simulink model "ddc_bpm_476_066"  (Simulink 7.8)
settings: Solver=ode45  StartTime=0.0  StopTime=2e-3  RelTol=1e-3
undefined symbols (not defined in the file): decim_factor_poly_35, dt_sim, frev_476, Fs_adc, n_ch, n_ovs, R_fofb, R_sec, R_sec_cfir, R_sec_pfir, xlipgetpartsetting
libraries: xbsIndex_r4 x1491, simulink x7
(part 7 of 12)

== system ddc_bpm_476_066/delta-sigma_monit/downsample8 ==
  din : Inport
  Down Sample : xbsIndex_r4/Down Sample  sample_ratio=R_fofb*R_sec_cfir*R_sec_pfir  sample_phase="Last Value of Frame  (most efficient)"  en=off  latency=1  dbl_ovrd=off  block_type=dsamp
  Down Sample5 : xbsIndex_r4/Down Sample  sample_ratio=R_sec*n_ovs  sample_phase="Last Value of Frame  (most efficient)"  en=off  latency=1  dbl_ovrd=off  block_type=dsamp
  dout : Outport
  wires:
  Down Sample5/1 -> Down Sample/1
  Down Sample/1 -> dout/1
  din/1 -> Down Sample5/1

== system ddc_bpm_476_066/delta-sigma_monit/fifo_tbt_q ==
  din : Inport
  re : Inport  Port=2
  we : Inport  Port=3
  clr_vld : Inport  Port=4
  From FIFO : xbsIndex_r4/From FIFO  shared_memory_name='fifo_monit_ds_q'  ownership=Owned elsewhere  performance_options=Standard_FIFO  depth=16  percent_nbits=1  has_arst=off  use_percent_full_port=off  gui_display_data_type=Fixed-point  arith_type="Signed  (2's comp)"  n_bits=26  bin_pt=22  preci_type=Single  dbl_ovrd=off  mem_type=Distributed RAM  block_type=fromfifo
      settings: AttributesFormatString=<< %<shared_memory_name> >>  infoedit=First-in-first-out (FIFO) block that reads FIFO data from shared memory storage.
  Inverter2 : xbsIndex_r4/Inverter  en=off  latency=0  dbl_ovrd=off  block_type=inv
  Inverter4 : xbsIndex_r4/Inverter  en=off  latency=0  dbl_ovrd=off  block_type=inv
  Logical : xbsIndex_r4/Logical  logical_function=AND  inputs=2  en=off  latency=0  precision=Full  arith_type=Unsigned  n_bits=16  bin_pt=0  align_bp=on  dbl_ovrd=off  block_type=logical
  Logical2 : xbsIndex_r4/Logical  logical_function=AND  inputs=2  en=off  latency=0  precision=Full  arith_type=Unsigned  n_bits=16  bin_pt=0  align_bp=on  dbl_ovrd=off  block_type=logical
  Register : xbsIndex_r4/Register  init=0  rst=off  en=off  dbl_ovrd=off  block_type=register
  ST11 : Subsystem
  ST2 : Subsystem
  ST7 : Subsystem
  To FIFO : xbsIndex_r4/To FIFO  shared_memory_name='fifo_monit_ds_q'  ownership=Locally owned  performance_options=Standard_FIFO  depth=16  percent_nbits=1  has_arst=off  use_percent_full_port=off  explicit_data_type=off  gui_display_data_type=Fixed-point  arith_type="Signed  (2's comp)"  n_bits=16  bin_pt=14  preci_type=Single  dbl_ovrd=off  mem_type=Distributed RAM  block_type=tofifo
      settings: AttributesFormatString=<< %<shared_memory_name> >>  infoedit=First-in-first-out (FIFO) block that writes FIFO data to shared memory storage.
  pulse_stretcher : Subsystem
  dout : Outport
  wr_full : Outport  Port=2
  rd_empty : Outport  Port=3
  valid_out : Outport  Port=4
  wires:
  Inverter2/1 -> Logical/2
  Logical/1 -> To FIFO/2, ST11/1(In)  "we"
  To FIFO/1 -> Inverter2/1, wr_full/1  "full"
  From FIFO/1 -> dout/1, ST2/1(In)  "dividend_data"
  we/1 -> Logical/1
  din/1 -> To FIFO/1
  From FIFO/2 -> rd_empty/1, Inverter4/1  "empty"
  clr_vld/1 -> pulse_stretcher/2(clr)  "clr"
  Register/1 -> pulse_stretcher/1(pulse_in)
  pulse_stretcher/1(extd_out) -> valid_out/1
  re/1 -> Logical2/1, ST7/1(In)
  Logical2/1 -> From FIFO/1, Register/1
  Inverter4/1 -> Logical2/2  "dividend_valid"

== system ddc_bpm_476_066/delta-sigma_monit/fifo_tbt_sum ==
  din : Inport
  re : Inport  Port=2
  we : Inport  Port=3
  clr_vld : Inport  Port=4
  From FIFO : xbsIndex_r4/From FIFO  shared_memory_name='fifo_monit_ds_sum'  ownership=Owned elsewhere  performance_options=Standard_FIFO  depth=16  percent_nbits=1  has_arst=off  use_percent_full_port=off  gui_display_data_type=Fixed-point  arith_type="Signed  (2's comp)"  n_bits=26  bin_pt=22  preci_type=Single  dbl_ovrd=off  mem_type=Distributed RAM  block_type=fromfifo
      settings: AttributesFormatString=<< %<shared_memory_name> >>  infoedit=First-in-first-out (FIFO) block that reads FIFO data from shared memory storage.
  Inverter2 : xbsIndex_r4/Inverter  en=off  latency=0  dbl_ovrd=off  block_type=inv
  Inverter4 : xbsIndex_r4/Inverter  en=off  latency=0  dbl_ovrd=off  block_type=inv
  Logical : xbsIndex_r4/Logical  logical_function=AND  inputs=2  en=off  latency=0  precision=Full  arith_type=Unsigned  n_bits=16  bin_pt=0  align_bp=on  dbl_ovrd=off  block_type=logical
  Logical2 : xbsIndex_r4/Logical  logical_function=AND  inputs=2  en=off  latency=0  precision=Full  arith_type=Unsigned  n_bits=16  bin_pt=0  align_bp=on  dbl_ovrd=off  block_type=logical
  Register : xbsIndex_r4/Register  init=0  rst=off  en=off  dbl_ovrd=off  block_type=register
  ST11 : Subsystem
  ST2 : Subsystem
  ST7 : Subsystem
  To FIFO : xbsIndex_r4/To FIFO  shared_memory_name='fifo_monit_ds_sum'  ownership=Locally owned  performance_options=Standard_FIFO  depth=16  percent_nbits=1  has_arst=off  use_percent_full_port=off  explicit_data_type=off  gui_display_data_type=Fixed-point  arith_type="Signed  (2's comp)"  n_bits=16  bin_pt=14  preci_type=Single  dbl_ovrd=off  mem_type=Distributed RAM  block_type=tofifo
      settings: AttributesFormatString=<< %<shared_memory_name> >>  infoedit=First-in-first-out (FIFO) block that writes FIFO data to shared memory storage.
  pulse_stretcher : Subsystem
  dout : Outport
  wr_full : Outport  Port=2
  rd_empty : Outport  Port=3
  valid_out : Outport  Port=4
  wires:
  Inverter2/1 -> Logical/2
  Logical/1 -> To FIFO/2, ST11/1(In)  "we"
  To FIFO/1 -> Inverter2/1, wr_full/1  "full"
  From FIFO/1 -> dout/1, ST2/1(In)  "dividend_data"
  we/1 -> Logical/1
  din/1 -> To FIFO/1
  From FIFO/2 -> rd_empty/1, Inverter4/1  "empty"
  clr_vld/1 -> pulse_stretcher/2(clr)  "clr"
  Register/1 -> pulse_stretcher/1(pulse_in)
  pulse_stretcher/1(extd_out) -> valid_out/1
  re/1 -> Logical2/1, ST7/1(In)
  Logical2/1 -> From FIFO/1, Register/1
  Inverter4/1 -> Logical2/2  "dividend_valid"

== system ddc_bpm_476_066/delta-sigma_monit/fifo_tbt_x ==
  din : Inport
  re : Inport  Port=2
  we : Inport  Port=3
  clr_vld : Inport  Port=4
  From FIFO : xbsIndex_r4/From FIFO  shared_memory_name='fifo_monit_ds_x'  ownership=Owned elsewhere  performance_options=Standard_FIFO  depth=16  percent_nbits=1  has_arst=off  use_percent_full_port=off  gui_display_data_type=Fixed-point  arith_type="Signed  (2's comp)"  n_bits=26  bin_pt=22  preci_type=Single  dbl_ovrd=off  mem_type=Distributed RAM  block_type=fromfifo
      settings: AttributesFormatString=<< %<shared_memory_name> >>  infoedit=First-in-first-out (FIFO) block that reads FIFO data from shared memory storage.
  Inverter2 : xbsIndex_r4/Inverter  en=off  latency=0  dbl_ovrd=off  block_type=inv
  Inverter4 : xbsIndex_r4/Inverter  en=off  latency=0  dbl_ovrd=off  block_type=inv
  Logical : xbsIndex_r4/Logical  logical_function=AND  inputs=2  en=off  latency=0  precision=Full  arith_type=Unsigned  n_bits=16  bin_pt=0  align_bp=on  dbl_ovrd=off  block_type=logical
  Logical2 : xbsIndex_r4/Logical  logical_function=AND  inputs=2  en=off  latency=0  precision=Full  arith_type=Unsigned  n_bits=16  bin_pt=0  align_bp=on  dbl_ovrd=off  block_type=logical
  Register : xbsIndex_r4/Register  init=0  rst=off  en=off  dbl_ovrd=off  block_type=register
  ST11 : Subsystem
  ST2 : Subsystem
  ST7 : Subsystem
  To FIFO : xbsIndex_r4/To FIFO  shared_memory_name='fifo_monit_ds_x'  ownership=Locally owned  performance_options=Standard_FIFO  depth=16  percent_nbits=1  has_arst=off  use_percent_full_port=off  explicit_data_type=off  gui_display_data_type=Fixed-point  arith_type="Signed  (2's comp)"  n_bits=16  bin_pt=14  preci_type=Single  dbl_ovrd=off  mem_type=Distributed RAM  block_type=tofifo
      settings: AttributesFormatString=<< %<shared_memory_name> >>  infoedit=First-in-first-out (FIFO) block that writes FIFO data to shared memory storage.
  pulse_stretcher : Subsystem
  dout : Outport
  wr_full : Outport  Port=2
  rd_empty : Outport  Port=3
  valid_out : Outport  Port=4
  wires:
  Inverter2/1 -> Logical/2
  Logical/1 -> To FIFO/2, ST11/1(In)  "we"
  To FIFO/1 -> Inverter2/1, wr_full/1  "full"
  From FIFO/1 -> dout/1, ST2/1(In)  "dividend_data"
  we/1 -> Logical/1
  din/1 -> To FIFO/1
  From FIFO/2 -> rd_empty/1, Inverter4/1  "empty"
  clr_vld/1 -> pulse_stretcher/2(clr)  "clr"
  Register/1 -> pulse_stretcher/1(pulse_in)
  pulse_stretcher/1(extd_out) -> valid_out/1
  re/1 -> Logical2/1, ST7/1(In)
  Logical2/1 -> From FIFO/1, Register/1
  Inverter4/1 -> Logical2/2  "dividend_valid"

== system ddc_bpm_476_066/delta-sigma_monit/fifo_tbt_y ==
  din : Inport
  re : Inport  Port=2
  we : Inport  Port=3
  clr_vld : Inport  Port=4
  From FIFO : xbsIndex_r4/From FIFO  shared_memory_name='fifo_monit_ds_y'  ownership=Owned elsewhere  performance_options=Standard_FIFO  depth=16  percent_nbits=1  has_arst=off  use_percent_full_port=off  gui_display_data_type=Fixed-point  arith_type="Signed  (2's comp)"  n_bits=26  bin_pt=22  preci_type=Single  dbl_ovrd=off  mem_type=Distributed RAM  block_type=fromfifo
      settings: AttributesFormatString=<< %<shared_memory_name> >>  infoedit=First-in-first-out (FIFO) block that reads FIFO data from shared memory storage.
  Inverter2 : xbsIndex_r4/Inverter  en=off  latency=0  dbl_ovrd=off  block_type=inv
  Inverter4 : xbsIndex_r4/Inverter  en=off  latency=0  dbl_ovrd=off  block_type=inv
  Logical : xbsIndex_r4/Logical  logical_function=AND  inputs=2  en=off  latency=0  precision=Full  arith_type=Unsigned  n_bits=16  bin_pt=0  align_bp=on  dbl_ovrd=off  block_type=logical
  Logical2 : xbsIndex_r4/Logical  logical_function=AND  inputs=2  en=off  latency=0  precision=Full  arith_type=Unsigned  n_bits=16  bin_pt=0  align_bp=on  dbl_ovrd=off  block_type=logical
  Register : xbsIndex_r4/Register  init=0  rst=off  en=off  dbl_ovrd=off  block_type=register
  ST11 : Subsystem
  ST2 : Subsystem
  ST7 : Subsystem
  To FIFO : xbsIndex_r4/To FIFO  shared_memory_name='fifo_monit_ds_y'  ownership=Locally owned  performance_options=Standard_FIFO  depth=16  percent_nbits=1  has_arst=off  use_percent_full_port=off  explicit_data_type=off  gui_display_data_type=Fixed-point  arith_type="Signed  (2's comp)"  n_bits=16  bin_pt=14  preci_type=Single  dbl_ovrd=off  mem_type=Distributed RAM  block_type=tofifo
      settings: AttributesFormatString=<< %<shared_memory_name> >>  infoedit=First-in-first-out (FIFO) block that writes FIFO data to shared memory storage.
  WaveScope : xbsIndex_r4/WaveScope  block_type=wavescope
  pulse_stretcher : Subsystem
  dout : Outport
  wr_full : Outport  Port=2
  rd_empty : Outport  Port=3
  valid_out : Outport  Port=4
  wires:
  Inverter2/1 -> Logical/2
  Logical/1 -> To FIFO/2, ST11/1(In)  "we"
  To FIFO/1 -> Inverter2/1, wr_full/1  "full"
  From FIFO/1 -> dout/1, ST2/1(In)  "dividend_data"
  we/1 -> Logical/1
  din/1 -> To FIFO/1
  From FIFO/2 -> rd_empty/1, Inverter4/1  "empty"
  clr_vld/1 -> pulse_stretcher/2(clr)  "clr"
  Register/1 -> pulse_stretcher/1(pulse_in)  "re_and_dly"
  pulse_stretcher/1(extd_out) -> valid_out/1  "vld_out"
  re/1 -> Logical2/1, ST7/1(In)  "re"
  Logical2/1 -> Register/1, From FIFO/1  "re_and"
  Inverter4/1 -> Logical2/2  "no_empty"

== system ddc_bpm_476_066/delta-sigma_monit/pulse_stretcher ==
  pulse_in : Inport
  clr : Inport  Port=2
  Inverter : xbsIndex_r4/Inverter  en=off  latency=0  dbl_ovrd=off  block_type=inv
  Logical1 : xbsIndex_r4/Logical  logical_function=AND  inputs=2  en=off  latency=0  precision=Full  arith_type=Unsigned  n_bits=16  bin_pt=0  align_bp=on  dbl_ovrd=off  block_type=logical
  Logical2 : xbsIndex_r4/Logical  logical_function=OR  inputs=2  en=off  latency=0  precision=Full  arith_type=Unsigned  n_bits=16  bin_pt=0  align_bp=on  dbl_ovrd=off  block_type=logical
  Logical3 : xbsIndex_r4/Logical  logical_function=OR  inputs=2  en=off  latency=0  precision=Full  arith_type=Unsigned  n_bits=16  bin_pt=0  align_bp=on  dbl_ovrd=off  block_type=logical
  Register : xbsIndex_r4/Register  init=0  rst=off  en=off  dbl_ovrd=off  block_type=register
  extd_out : Outport
  wires:
  Register/1 -> Logical1/1, Logical3/2
  clr/1 -> Inverter/1
  Logical1/1 -> Logical2/2
  Logical2/1 -> Register/1
  Inverter/1 -> Logical1/2
  Logical3/1 -> extd_out/1
  pulse_in/1 -> Logical3/1, Logical2/1

== system ddc_bpm_476_066/delta-sigma_monit/pulse_stretcher1 ==
  pulse_in : Inport
  clr : Inport  Port=2
  Inverter : xbsIndex_r4/Inverter  en=off  latency=0  dbl_ovrd=off  block_type=inv
  Logical1 : xbsIndex_r4/Logical  logical_function=AND  inputs=2  en=off  latency=0  precision=Full  arith_type=Unsigned  n_bits=16  bin_pt=0  align_bp=on  dbl_ovrd=off  block_type=logical
  Logical2 : xbsIndex_r4/Logical  logical_function=OR  inputs=2  en=off  latency=0  precision=Full  arith_type=Unsigned  n_bits=16  bin_pt=0  align_bp=on  dbl_ovrd=off  block_type=logical
  Logical3 : xbsIndex_r4/Logical  logical_function=OR  inputs=2  en=off  latency=0  precision=Full  arith_type=Unsigned  n_bits=16  bin_pt=0  align_bp=on  dbl_ovrd=off  block_type=logical
  Register : xbsIndex_r4/Register  init=0  rst=off  en=off  dbl_ovrd=off  block_type=register
  extd_out : Outport
  wires:
  Register/1 -> Logical1/1, Logical3/2
  clr/1 -> Inverter/1
  Logical1/1 -> Logical2/2
  Logical2/1 -> Register/1
  Inverter/1 -> Logical1/2
  Logical3/1 -> extd_out/1
  pulse_in/1 -> Logical3/1, Logical2/1

== system ddc_bpm_476_066/delta-sigma_monit/pulse_stretcher2 ==
  pulse_in : Inport
  clr : Inport  Port=2
  Inverter : xbsIndex_r4/Inverter  en=off  latency=0  dbl_ovrd=off  block_type=inv
  Logical1 : xbsIndex_r4/Logical  logical_function=AND  inputs=2  en=off  latency=0  precision=Full  arith_type=Unsigned  n_bits=16  bin_pt=0  align_bp=on  dbl_ovrd=off  block_type=logical
  Logical2 : xbsIndex_r4/Logical  logical_function=OR  inputs=2  en=off  latency=0  precision=Full  arith_type=Unsigned  n_bits=16  bin_pt=0  align_bp=on  dbl_ovrd=off  block_type=logical
  Logical3 : xbsIndex_r4/Logical  logical_function=OR  inputs=2  en=off  latency=0  precision=Full  arith_type=Unsigned  n_bits=16  bin_pt=0  align_bp=on  dbl_ovrd=off  block_type=logical
  Register : xbsIndex_r4/Register  init=0  rst=off  en=off  dbl_ovrd=off  block_type=register
  extd_out : Outport
  wires:
  Register/1 -> Logical1/1, Logical3/2
  clr/1 -> Inverter/1
  Logical1/1 -> Logical2/2
  Logical2/1 -> Register/1
  Inverter/1 -> Logical1/2
  Logical3/1 -> extd_out/1
  pulse_in/1 -> Logical3/1, Logical2/1

== system ddc_bpm_476_066/delta-sigma_monit/pulse_stretcher3 ==
  pulse_in : Inport
  clr : Inport  Port=2
  Inverter : xbsIndex_r4/Inverter  en=off  latency=0  dbl_ovrd=off  block_type=inv
  Logical1 : xbsIndex_r4/Logical  logical_function=AND  inputs=2  en=off  latency=0  precision=Full  arith_type=Unsigned  n_bits=16  bin_pt=0  align_bp=on  dbl_ovrd=off  block_type=logical
  Logical2 : xbsIndex_r4/Logical  logical_function=OR  inputs=2  en=off  latency=0  precision=Full  arith_type=Unsigned  n_bits=16  bin_pt=0  align_bp=on  dbl_ovrd=off  block_type=logical
  Logical3 : xbsIndex_r4/Logical  logical_function=OR  inputs=2  en=off  latency=0  precision=Full  arith_type=Unsigned  n_bits=16  bin_pt=0  align_bp=on  dbl_ovrd=off  block_type=logical
  Register : xbsIndex_r4/Register  init=0  rst=off  en=off  dbl_ovrd=off  block_type=register
  extd_out : Outport
  wires:
  Register/1 -> Logical1/1, Logical3/2
  clr/1 -> Inverter/1
  Logical1/1 -> Logical2/2
  Logical2/1 -> Register/1
  Inverter/1 -> Logical1/2
  Logical3/1 -> extd_out/1
  pulse_in/1 -> Logical3/1, Logical2/1

== system ddc_bpm_476_066/delta-sigma_tbt/DataReg_En ==
  Din : Inport
  en : Inport  Port=2
  Register : xbsIndex_r4/Register  init=0  rst=off  en=on  dbl_ovrd=off  block_type=register
      settings: block_version=VER_STRING_GOES_HERE
  Register1 : xbsIndex_r4/Register  init=0  rst=off  en=off  dbl_ovrd=off  block_type=register
      settings: block_version=VER_STRING_GOES_HERE
  Dout : Outport
  Valid : Outport  Port=2
  wires:
  Din/1 -> Register/1
  Register/1 -> Dout/1
  Register1/1 -> Valid/1
  en/1 -> Register1/1, Register/2

== system ddc_bpm_476_066/delta-sigma_tbt/DataReg_En1 ==
  Din : Inport
  en : Inport  Port=2
  Register : xbsIndex_r4/Register  init=0  rst=off  en=on  dbl_ovrd=off  block_type=register
      settings: block_version=VER_STRING_GOES_HERE
  Register1 : xbsIndex_r4/Register  init=0  rst=off  en=off  dbl_ovrd=off  block_type=register
      settings: block_version=VER_STRING_GOES_HERE
  Dout : Outport
  Valid : Outport  Port=2
  wires:
  Din/1 -> Register/1
  Register/1 -> Dout/1
  Register1/1 -> Valid/1
  en/1 -> Register1/1, Register/2

== system ddc_bpm_476_066/delta-sigma_tbt/DataReg_En2 ==
  Din : Inport
  en : Inport  Port=2
  Register : xbsIndex_r4/Register  init=0  rst=off  en=on  dbl_ovrd=off  block_type=register
      settings: block_version=VER_STRING_GOES_HERE
  Register1 : xbsIndex_r4/Register  init=0  rst=off  en=off  dbl_ovrd=off  block_type=register
      settings: block_version=VER_STRING_GOES_HERE
  Dout : Outport
  Valid : Outport  Port=2
  wires:
  Din/1 -> Register/1
  Register/1 -> Dout/1
  Register1/1 -> Valid/1
  en/1 -> Register1/1, Register/2

== system ddc_bpm_476_066/delta-sigma_tbt/DataReg_En3 ==
  Din : Inport
  en : Inport  Port=2
  Register : xbsIndex_r4/Register  init=0  rst=off  en=on  dbl_ovrd=off  block_type=register
      settings: block_version=VER_STRING_GOES_HERE
  Register1 : xbsIndex_r4/Register  init=0  rst=off  en=off  dbl_ovrd=off  block_type=register
      settings: block_version=VER_STRING_GOES_HERE
  Dout : Outport
  Valid : Outport  Port=2
  wires:
  Din/1 -> Register/1
  Register/1 -> Dout/1
  Register1/1 -> Valid/1
  en/1 -> Register1/1, Register/2

== system ddc_bpm_476_066/delta-sigma_tbt/ST1 ==
  In : Inport
  Display : Display
  Sample Time : xbsIndex_r4/Sample Time  block_type=sampletime
      settings: infoedit="The Sample Time block reports the normalized sample period of its input.  A signal's normalized sample period is not equivalent to its Simulink absolute sample period.<br><br>Hardware notes: This block is implemented as a constant in hardware."
  X_monit1 : xbsIndex_r4/Gateway Out  inherit_from_input=on  hdl_port=off  timing_constraint=Data Rate  locs_specified=off  LOCs={}  UseAsDAC=off  DACChannel='1'  block_type=gatewayout
      settings: infoedit="Gateway out block.  Converts Xilinx fixed-point or floating-point type inputs into ouputs of type Simulink integer, single, double, or fixed point.<br><br>Hardware notes:  In hardware these blocks become top level output ports or are discarded, depending on how they are configured."
  wires:
  X_monit1/1 -> Display/1
  Sample Time/1 -> X_monit1/1
  In/1 -> Sample Time/1

== system ddc_bpm_476_066/delta-sigma_tbt/ST2 ==
  In : Inport
  Display : Display
  Sample Time : xbsIndex_r4/Sample Time  block_type=sampletime
      settings: infoedit="The Sample Time block reports the normalized sample period of its input.  A signal's normalized sample period is not equivalent to its Simulink absolute sample period.<br><br>Hardware notes: This block is implemented as a constant in hardware."
  X_monit1 : xbsIndex_r4/Gateway Out  inherit_from_input=on  hdl_port=off  timing_constraint=Data Rate  locs_specified=off  LOCs={}  UseAsDAC=off  DACChannel='1'  block_type=gatewayout
      settings: infoedit="Gateway out block.  Converts Xilinx fixed-point or floating-point type inputs into ouputs of type Simulink integer, single, double, or fixed point.<br><br>Hardware notes:  In hardware these blocks become top level output ports or are discarded, depending on how they are configured."
  wires:
  X_monit1/1 -> Display/1
  Sample Time/1 -> X_monit1/1
  In/1 -> Sample Time/1

== system ddc_bpm_476_066/delta-sigma_tbt/ST3 ==
  In : Inport
  Display : Display
  Sample Time : xbsIndex_r4/Sample Time  block_type=sampletime
      settings: infoedit="The Sample Time block reports the normalized sample period of its input.  A signal's normalized sample period is not equivalent to its Simulink absolute sample period.<br><br>Hardware notes: This block is implemented as a constant in hardware."
  X_monit1 : xbsIndex_r4/Gateway Out  inherit_from_input=on  hdl_port=off  timing_constraint=Data Rate  locs_specified=off  LOCs={}  UseAsDAC=off  DACChannel='1'  block_type=gatewayout
      settings: infoedit="Gateway out block.  Converts Xilinx fixed-point or floating-point type inputs into ouputs of type Simulink integer, single, double, or fixed point.<br><br>Hardware notes:  In hardware these blocks become top level output ports or are discarded, depending on how they are configured."
  wires:
  X_monit1/1 -> Display/1
  Sample Time/1 -> X_monit1/1
  In/1 -> Sample Time/1

== system ddc_bpm_476_066/delta-sigma_tbt/ST4 ==
  In : Inport
  Display : Display
  Sample Time : xbsIndex_r4/Sample Time  block_type=sampletime
      settings: infoedit="The Sample Time block reports the normalized sample period of its input.  A signal's normalized sample period is not equivalent to its Simulink absolute sample period.<br><br>Hardware notes: This block is implemented as a constant in hardware."
  X_monit1 : xbsIndex_r4/Gateway Out  inherit_from_input=on  hdl_port=off  timing_constraint=Data Rate  locs_specified=off  LOCs={}  UseAsDAC=off  DACChannel='1'  block_type=gatewayout
      settings: infoedit="Gateway out block.  Converts Xilinx fixed-point or floating-point type inputs into ouputs of type Simulink integer, single, double, or fixed point.<br><br>Hardware notes:  In hardware these blocks become top level output ports or are discarded, depending on how they are configured."
  wires:
  X_monit1/1 -> Display/1
  Sample Time/1 -> X_monit1/1
  In/1 -> Sample Time/1

== system ddc_bpm_476_066/delta-sigma_tbt/ST5 ==
  In : Inport
  Display : Display
  Sample Time : xbsIndex_r4/Sample Time  block_type=sampletime
      settings: infoedit="The Sample Time block reports the normalized sample period of its input.  A signal's normalized sample period is not equivalent to its Simulink absolute sample period.<br><br>Hardware notes: This block is implemented as a constant in hardware."
  X_monit1 : xbsIndex_r4/Gateway Out  inherit_from_input=on  hdl_port=off  timing_constraint=Data Rate  locs_specified=off  LOCs={}  UseAsDAC=off  DACChannel='1'  block_type=gatewayout
      settings: infoedit="Gateway out block.  Converts Xilinx fixed-point or floating-point type inputs into ouputs of type Simulink integer, single, double, or fixed point.<br><br>Hardware notes:  In hardware these blocks become top level output ports or are discarded, depending on how they are configured."
  wires:
  X_monit1/1 -> Display/1
  Sample Time/1 -> X_monit1/1
  In/1 -> Sample Time/1

== system ddc_bpm_476_066/delta-sigma_tbt/ST6 ==
  In : Inport
  Display : Display
  Sample Time : xbsIndex_r4/Sample Time  block_type=sampletime
      settings: infoedit="The Sample Time block reports the normalized sample period of its input.  A signal's normalized sample period is not equivalent to its Simulink absolute sample period.<br><br>Hardware notes: This block is implemented as a constant in hardware."
  X_monit1 : xbsIndex_r4/Gateway Out  inherit_from_input=on  hdl_port=off  timing_constraint=Data Rate  locs_specified=off  LOCs={}  UseAsDAC=off  DACChannel='1'  block_type=gatewayout
      settings: infoedit="Gateway out block.  Converts Xilinx fixed-point or floating-point type inputs into ouputs of type Simulink integer, single, double, or fixed point.<br><br>Hardware notes:  In hardware these blocks become top level output ports or are discarded, depending on how they are configured."
  wires:
  X_monit1/1 -> Display/1
  Sample Time/1 -> X_monit1/1
  In/1 -> Sample Time/1

== system ddc_bpm_476_066/delta-sigma_tbt/ST7 ==
  In : Inport
  Display : Display
  Sample Time : xbsIndex_r4/Sample Time  block_type=sampletime
      settings: infoedit="The Sample Time block reports the normalized sample period of its input.  A signal's normalized sample period is not equivalent to its Simulink absolute sample period.<br><br>Hardware notes: This block is implemented as a constant in hardware."
  X_monit1 : xbsIndex_r4/Gateway Out  inherit_from_input=on  hdl_port=off  timing_constraint=Data Rate  locs_specified=off  LOCs={}  UseAsDAC=off  DACChannel='1'  block_type=gatewayout
      settings: infoedit="Gateway out block.  Converts Xilinx fixed-point or floating-point type inputs into ouputs of type Simulink integer, single, double, or fixed point.<br><br>Hardware notes:  In hardware these blocks become top level output ports or are discarded, depending on how they are configured."
  wires:
  X_monit1/1 -> Display/1
  Sample Time/1 -> X_monit1/1
  In/1 -> Sample Time/1

== system ddc_bpm_476_066/delta-sigma_tbt/ST8 ==
  In : Inport
  Display : Display
  Sample Time : xbsIndex_r4/Sample Time  block_type=sampletime
      settings: infoedit="The Sample Time block reports the normalized sample period of its input.  A signal's normalized sample period is not equivalent to its Simulink absolute sample period.<br><br>Hardware notes: This block is implemented as a constant in hardware."
  X_monit1 : xbsIndex_r4/Gateway Out  inherit_from_input=on  hdl_port=off  timing_constraint=Data Rate  locs_specified=off  LOCs={}  UseAsDAC=off  DACChannel='1'  block_type=gatewayout
      settings: infoedit="Gateway out block.  Converts Xilinx fixed-point or floating-point type inputs into ouputs of type Simulink integer, single, double, or fixed point.<br><br>Hardware notes:  In hardware these blocks become top level output ports or are discarded, depending on how they are configured."
  wires:
  X_monit1/1 -> Display/1
  Sample Time/1 -> X_monit1/1
  In/1 -> Sample Time/1

== system ddc_bpm_476_066/delta-sigma_tbt/ST9 ==
  In : Inport
  Display : Display
  Sample Time : xbsIndex_r4/Sample Time  block_type=sampletime
      settings: infoedit="The Sample Time block reports the normalized sample period of its input.  A signal's normalized sample period is not equivalent to its Simulink absolute sample period.<br><br>Hardware notes: This block is implemented as a constant in hardware."
  X_monit1 : xbsIndex_r4/Gateway Out  inherit_from_input=on  hdl_port=off  timing_constraint=Data Rate  locs_specified=off  LOCs={}  UseAsDAC=off  DACChannel='1'  block_type=gatewayout
      settings: infoedit="Gateway out block.  Converts Xilinx fixed-point or floating-point type inputs into ouputs of type Simulink integer, single, double, or fixed point.<br><br>Hardware notes:  In hardware these blocks become top level output ports or are discarded, depending on how they are configured."
  wires:
  X_monit1/1 -> Display/1
  Sample Time/1 -> X_monit1/1
  In/1 -> Sample Time/1

== system ddc_bpm_476_066/delta-sigma_tbt/fifo_tbt_q ==
  din : Inport
  re : Inport  Port=2
  we : Inport  Port=3
  clr_vld : Inport  Port=4
  From FIFO : xbsIndex_r4/From FIFO  shared_memory_name='fifo_tbt_ds_q'  ownership=Owned elsewhere  performance_options=Standard_FIFO  depth=16  percent_nbits=1  has_arst=off  use_percent_full_port=off  gui_display_data_type=Fixed-point  arith_type="Signed  (2's comp)"  n_bits=26  bin_pt=22  preci_type=Single  dbl_ovrd=off  mem_type=Distributed RAM  block_type=fromfifo
      settings: AttributesFormatString=<< %<shared_memory_name> >>  infoedit=First-in-first-out (FIFO) block that reads FIFO data from shared memory storage.
  Inverter2 : xbsIndex_r4/Inverter  en=off  latency=0  dbl_ovrd=off  block_type=inv
  Inverter4 : xbsIndex_r4/Inverter  en=off  latency=0  dbl_ovrd=off  block_type=inv
  Logical : xbsIndex_r4/Logical  logical_function=AND  inputs=2  en=off  latency=0  precision=Full  arith_type=Unsigned  n_bits=16  bin_pt=0  align_bp=on  dbl_ovrd=off  block_type=logical
  Logical2 : xbsIndex_r4/Logical  logical_function=AND  inputs=2  en=off  latency=0  precision=Full  arith_type=Unsigned  n_bits=16  bin_pt=0  align_bp=on  dbl_ovrd=off  block_type=logical
  Register : xbsIndex_r4/Register  init=0  rst=off  en=off  dbl_ovrd=off  block_type=register
  ST11 : Subsystem
  ST2 : Subsystem
  ST7 : Subsystem
  To FIFO : xbsIndex_r4/To FIFO  shared_memory_name='fifo_tbt_ds_q'  ownership=Locally owned  performance_options=Standard_FIFO  depth=16  percent_nbits=1  has_arst=off  use_percent_full_port=off  explicit_data_type=off  gui_display_data_type=Fixed-point  arith_type="Signed  (2's comp)"  n_bits=16  bin_pt=14  preci_type=Single  dbl_ovrd=off  mem_type=Distributed RAM  block_type=tofifo
      settings: AttributesFormatString=<< %<shared_memory_name> >>  infoedit=First-in-first-out (FIFO) block that writes FIFO data to shared memory storage.
  pulse_stretcher : Subsystem
  dout : Outport
  wr_full : Outport  Port=2
  rd_empty : Outport  Port=3
  valid_out : Outport  Port=4
  wires:
  Inverter2/1 -> Logical/2
  Logical/1 -> To FIFO/2, ST11/1(In)  "we"
  To FIFO/1 -> Inverter2/1, wr_full/1  "full"
  From FIFO/1 -> dout/1, ST2/1(In)  "dividend_data"
  we/1 -> Logical/1
  din/1 -> To FIFO/1
  From FIFO/2 -> rd_empty/1, Inverter4/1  "empty"
  clr_vld/1 -> pulse_stretcher/2(clr)  "clr"
  Register/1 -> pulse_stretcher/1(pulse_in)
  pulse_stretcher/1(extd_out) -> valid_out/1
  re/1 -> Logical2/1, ST7/1(In)
  Logical2/1 -> From FIFO/1, Register/1
  Inverter4/1 -> Logical2/2  "dividend_valid"

== system ddc_bpm_476_066/delta-sigma_tbt/fifo_tbt_sum ==
  din : Inport
  re : Inport  Port=2
  we : Inport  Port=3
  clr_vld : Inport  Port=4
  From FIFO : xbsIndex_r4/From FIFO  shared_memory_name='fifo_tbt_ds_sum'  ownership=Owned elsewhere  performance_options=Standard_FIFO  depth=16  percent_nbits=1  has_arst=off  use_percent_full_port=off  gui_display_data_type=Fixed-point  arith_type="Signed  (2's comp)"  n_bits=26  bin_pt=22  preci_type=Single  dbl_ovrd=off  mem_type=Distributed RAM  block_type=fromfifo
      settings: AttributesFormatString=<< %<shared_memory_name> >>  infoedit=First-in-first-out (FIFO) block that reads FIFO data from shared memory storage.
  Inverter2 : xbsIndex_r4/Inverter  en=off  latency=0  dbl_ovrd=off  block_type=inv
  Inverter4 : xbsIndex_r4/Inverter  en=off  latency=0  dbl_ovrd=off  block_type=inv
  Logical : xbsIndex_r4/Logical  logical_function=AND  inputs=2  en=off  latency=0  precision=Full  arith_type=Unsigned  n_bits=16  bin_pt=0  align_bp=on  dbl_ovrd=off  block_type=logical
  Logical2 : xbsIndex_r4/Logical  logical_function=AND  inputs=2  en=off  latency=0  precision=Full  arith_type=Unsigned  n_bits=16  bin_pt=0  align_bp=on  dbl_ovrd=off  block_type=logical
  Register : xbsIndex_r4/Register  init=0  rst=off  en=off  dbl_ovrd=off  block_type=register
  ST11 : Subsystem
  ST2 : Subsystem
  ST7 : Subsystem
  To FIFO : xbsIndex_r4/To FIFO  shared_memory_name='fifo_tbt_ds_sum'  ownership=Locally owned  performance_options=Standard_FIFO  depth=16  percent_nbits=1  has_arst=off  use_percent_full_port=off  explicit_data_type=off  gui_display_data_type=Fixed-point  arith_type="Signed  (2's comp)"  n_bits=16  bin_pt=14  preci_type=Single  dbl_ovrd=off  mem_type=Distributed RAM  block_type=tofifo
      settings: AttributesFormatString=<< %<shared_memory_name> >>  infoedit=First-in-first-out (FIFO) block that writes FIFO data to shared memory storage.
  pulse_stretcher : Subsystem
  dout : Outport
  wr_full : Outport  Port=2
  rd_empty : Outport  Port=3
  valid_out : Outport  Port=4
  wires:
  Inverter2/1 -> Logical/2
  Logical/1 -> To FIFO/2, ST11/1(In)  "we"
  To FIFO/1 -> Inverter2/1, wr_full/1  "full"
  From FIFO/1 -> dout/1, ST2/1(In)  "dividend_data"
  we/1 -> Logical/1
  din/1 -> To FIFO/1
  From FIFO/2 -> rd_empty/1, Inverter4/1  "empty"
  clr_vld/1 -> pulse_stretcher/2(clr)  "clr"
  Register/1 -> pulse_stretcher/1(pulse_in)
  pulse_stretcher/1(extd_out) -> valid_out/1
  re/1 -> Logical2/1, ST7/1(In)
  Logical2/1 -> From FIFO/1, Register/1
  Inverter4/1 -> Logical2/2  "dividend_valid"

== system ddc_bpm_476_066/delta-sigma_tbt/fifo_tbt_x ==
  din : Inport
  re : Inport  Port=2
  we : Inport  Port=3
  clr_vld : Inport  Port=4
  From FIFO : xbsIndex_r4/From FIFO  shared_memory_name='fifo_tbt_ds_x'  ownership=Owned elsewhere  performance_options=Standard_FIFO  depth=16  percent_nbits=1  has_arst=off  use_percent_full_port=off  gui_display_data_type=Fixed-point  arith_type="Signed  (2's comp)"  n_bits=26  bin_pt=22  preci_type=Single  dbl_ovrd=off  mem_type=Distributed RAM  block_type=fromfifo
      settings: AttributesFormatString=<< %<shared_memory_name> >>  infoedit=First-in-first-out (FIFO) block that reads FIFO data from shared memory storage.
  Inverter2 : xbsIndex_r4/Inverter  en=off  latency=0  dbl_ovrd=off  block_type=inv
  Inverter4 : xbsIndex_r4/Inverter  en=off  latency=0  dbl_ovrd=off  block_type=inv
  Logical : xbsIndex_r4/Logical  logical_function=AND  inputs=2  en=off  latency=0  precision=Full  arith_type=Unsigned  n_bits=16  bin_pt=0  align_bp=on  dbl_ovrd=off  block_type=logical
  Logical2 : xbsIndex_r4/Logical  logical_function=AND  inputs=2  en=off  latency=0  precision=Full  arith_type=Unsigned  n_bits=16  bin_pt=0  align_bp=on  dbl_ovrd=off  block_type=logical
  Register : xbsIndex_r4/Register  init=0  rst=off  en=off  dbl_ovrd=off  block_type=register
  ST11 : Subsystem
  ST2 : Subsystem
  ST7 : Subsystem
  To FIFO : xbsIndex_r4/To FIFO  shared_memory_name='fifo_tbt_ds_x'  ownership=Locally owned  performance_options=Standard_FIFO  depth=16  percent_nbits=1  has_arst=off  use_percent_full_port=off  explicit_data_type=off  gui_display_data_type=Fixed-point  arith_type="Signed  (2's comp)"  n_bits=16  bin_pt=14  preci_type=Single  dbl_ovrd=off  mem_type=Distributed RAM  block_type=tofifo
      settings: AttributesFormatString=<< %<shared_memory_name> >>  infoedit=First-in-first-out (FIFO) block that writes FIFO data to shared memory storage.
  pulse_stretcher : Subsystem
  dout : Outport
  wr_full : Outport  Port=2
  rd_empty : Outport  Port=3
  valid_out : Outport  Port=4
  wires:
  Inverter2/1 -> Logical/2
  Logical/1 -> To FIFO/2, ST11/1(In)  "we"
  To FIFO/1 -> Inverter2/1, wr_full/1  "full"
  From FIFO/1 -> dout/1, ST2/1(In)  "dividend_data"
  we/1 -> Logical/1
  din/1 -> To FIFO/1
  From FIFO/2 -> rd_empty/1, Inverter4/1  "empty"
  clr_vld/1 -> pulse_stretcher/2(clr)  "clr"
  Register/1 -> pulse_stretcher/1(pulse_in)
  pulse_stretcher/1(extd_out) -> valid_out/1
  re/1 -> Logical2/1, ST7/1(In)
  Logical2/1 -> From FIFO/1, Register/1
  Inverter4/1 -> Logical2/2  "dividend_valid"

== system ddc_bpm_476_066/delta-sigma_tbt/fifo_tbt_y ==
  din : Inport
  re : Inport  Port=2
  we : Inport  Port=3
  clr_vld : Inport  Port=4
  From FIFO : xbsIndex_r4/From FIFO  shared_memory_name='fifo_tbt_ds_y'  ownership=Owned elsewhere  performance_options=Standard_FIFO  depth=16  percent_nbits=1  has_arst=off  use_percent_full_port=off  gui_display_data_type=Fixed-point  arith_type="Signed  (2's comp)"  n_bits=26  bin_pt=22  preci_type=Single  dbl_ovrd=off  mem_type=Distributed RAM  block_type=fromfifo
      settings: AttributesFormatString=<< %<shared_memory_name> >>  infoedit=First-in-first-out (FIFO) block that reads FIFO data from shared memory storage.
  Inverter2 : xbsIndex_r4/Inverter  en=off  latency=0  dbl_ovrd=off  block_type=inv
  Inverter4 : xbsIndex_r4/Inverter  en=off  latency=0  dbl_ovrd=off  block_type=inv
  Logical : xbsIndex_r4/Logical  logical_function=AND  inputs=2  en=off  latency=0  precision=Full  arith_type=Unsigned  n_bits=16  bin_pt=0  align_bp=on  dbl_ovrd=off  block_type=logical
  Logical2 : xbsIndex_r4/Logical  logical_function=AND  inputs=2  en=off  latency=0  precision=Full  arith_type=Unsigned  n_bits=16  bin_pt=0  align_bp=on  dbl_ovrd=off  block_type=logical
  Register : xbsIndex_r4/Register  init=0  rst=off  en=off  dbl_ovrd=off  block_type=register
  ST11 : Subsystem
  ST2 : Subsystem
  ST7 : Subsystem
  To FIFO : xbsIndex_r4/To FIFO  shared_memory_name='fifo_tbt_ds_y'  ownership=Locally owned  performance_options=Standard_FIFO  depth=16  percent_nbits=1  has_arst=off  use_percent_full_port=off  explicit_data_type=off  gui_display_data_type=Fixed-point  arith_type="Signed  (2's comp)"  n_bits=16  bin_pt=14  preci_type=Single  dbl_ovrd=off  mem_type=Distributed RAM  block_type=tofifo
      settings: AttributesFormatString=<< %<shared_memory_name> >>  infoedit=First-in-first-out (FIFO) block that writes FIFO data to shared memory storage.
  WaveScope : xbsIndex_r4/WaveScope  block_type=wavescope
  pulse_stretcher : Subsystem
  dout : Outport
  wr_full : Outport  Port=2
  rd_empty : Outport  Port=3
  valid_out : Outport  Port=4
  wires:
  Inverter2/1 -> Logical/2
  Logical/1 -> To FIFO/2, ST11/1(In)  "we"
  To FIFO/1 -> Inverter2/1, wr_full/1  "full"
  From FIFO/1 -> dout/1, ST2/1(In)  "dividend_data"
  we/1 -> Logical/1
  din/1 -> To FIFO/1
  From FIFO/2 -> rd_empty/1, Inverter4/1  "empty"
  clr_vld/1 -> pulse_stretcher/2(clr)  "clr"
  Register/1 -> pulse_stretcher/1(pulse_in)  "re_and_dly"
  pulse_stretcher/1(extd_out) -> valid_out/1  "vld_out"
  re/1 -> Logical2/1, ST7/1(In)  "re"
  Logical2/1 -> Register/1, From FIFO/1  "re_and"
  Inverter4/1 -> Logical2/2  "no_empty"

== system ddc_bpm_476_066/delta-sigma_tbt/pulse_stretcher ==
  pulse_in : Inport
  clr : Inport  Port=2
  Inverter : xbsIndex_r4/Inverter  en=off  latency=0  dbl_ovrd=off  block_type=inv
  Logical1 : xbsIndex_r4/Logical  logical_function=AND  inputs=2  en=off  latency=0  precision=Full  arith_type=Unsigned  n_bits=16  bin_pt=0  align_bp=on  dbl_ovrd=off  block_type=logical
  Logical2 : xbsIndex_r4/Logical  logical_function=OR  inputs=2  en=off  latency=0  precision=Full  arith_type=Unsigned  n_bits=16  bin_pt=0  align_bp=on  dbl_ovrd=off  block_type=logical
  Logical3 : xbsIndex_r4/Logical  logical_function=OR  inputs=2  en=off  latency=0  precision=Full  arith_type=Unsigned  n_bits=16  bin_pt=0  align_bp=on  dbl_ovrd=off  block_type=logical
  Register : xbsIndex_r4/Register  init=0  rst=off  en=off  dbl_ovrd=off  block_type=register
  extd_out : Outport
  wires:
  Register/1 -> Logical1/1, Logical3/2
  clr/1 -> Inverter/1
  Logical1/1 -> Logical2/2
  Logical2/1 -> Register/1
  Inverter/1 -> Logical1/2
  Logical3/1 -> extd_out/1
  pulse_in/1 -> Logical3/1, Logical2/1

== system ddc_bpm_476_066/delta-sigma_tbt/pulse_stretcher1 ==
  pulse_in : Inport
  clr : Inport  Port=2
  Inverter : xbsIndex_r4/Inverter  en=off  latency=0  dbl_ovrd=off  block_type=inv
  Logical1 : xbsIndex_r4/Logical  logical_function=AND  inputs=2  en=off  latency=0  precision=Full  arith_type=Unsigned  n_bits=16  bin_pt=0  align_bp=on  dbl_ovrd=off  block_type=logical
  Logical2 : xbsIndex_r4/Logical  logical_function=OR  inputs=2  en=off  latency=0  precision=Full  arith_type=Unsigned  n_bits=16  bin_pt=0  align_bp=on  dbl_ovrd=off  block_type=logical
  Logical3 : xbsIndex_r4/Logical  logical_function=OR  inputs=2  en=off  latency=0  precision=Full  arith_type=Unsigned  n_bits=16  bin_pt=0  align_bp=on  dbl_ovrd=off  block_type=logical
  Register : xbsIndex_r4/Register  init=0  rst=off  en=off  dbl_ovrd=off  block_type=register
  extd_out : Outport
  wires:
  Register/1 -> Logical1/1, Logical3/2
  clr/1 -> Inverter/1
  Logical1/1 -> Logical2/2
  Logical2/1 -> Register/1
  Inverter/1 -> Logical1/2
  Logical3/1 -> extd_out/1
  pulse_in/1 -> Logical3/1, Logical2/1

== system ddc_bpm_476_066/delta-sigma_tbt/pulse_stretcher2 ==
  pulse_in : Inport
  clr : Inport  Port=2
  Inverter : xbsIndex_r4/Inverter  en=off  latency=0  dbl_ovrd=off  block_type=inv
  Logical1 : xbsIndex_r4/Logical  logical_function=AND  inputs=2  en=off  latency=0  precision=Full  arith_type=Unsigned  n_bits=16  bin_pt=0  align_bp=on  dbl_ovrd=off  block_type=logical
  Logical2 : xbsIndex_r4/Logical  logical_function=OR  inputs=2  en=off  latency=0  precision=Full  arith_type=Unsigned  n_bits=16  bin_pt=0  align_bp=on  dbl_ovrd=off  block_type=logical
  Logical3 : xbsIndex_r4/Logical  logical_function=OR  inputs=2  en=off  latency=0  precision=Full  arith_type=Unsigned  n_bits=16  bin_pt=0  align_bp=on  dbl_ovrd=off  block_type=logical
  Register : xbsIndex_r4/Register  init=0  rst=off  en=off  dbl_ovrd=off  block_type=register
  extd_out : Outport
  wires:
  Register/1 -> Logical1/1, Logical3/2
  clr/1 -> Inverter/1
  Logical1/1 -> Logical2/2
  Logical2/1 -> Register/1
  Inverter/1 -> Logical1/2
  Logical3/1 -> extd_out/1
  pulse_in/1 -> Logical3/1, Logical2/1

== system ddc_bpm_476_066/delta-sigma_tbt/pulse_stretcher3 ==
  pulse_in : Inport
  clr : Inport  Port=2
  Inverter : xbsIndex_r4/Inverter  en=off  latency=0  dbl_ovrd=off  block_type=inv
  Logical1 : xbsIndex_r4/Logical  logical_function=AND  inputs=2  en=off  latency=0  precision=Full  arith_type=Unsigned  n_bits=16  bin_pt=0  align_bp=on  dbl_ovrd=off  block_type=logical
  Logical2 : xbsIndex_r4/Logical  logical_function=OR  inputs=2  en=off  latency=0  precision=Full  arith_type=Unsigned  n_bits=16  bin_pt=0  align_bp=on  dbl_ovrd=off  block_type=logical
  Logical3 : xbsIndex_r4/Logical  logical_function=OR  inputs=2  en=off  latency=0  precision=Full  arith_type=Unsigned  n_bits=16  bin_pt=0  align_bp=on  dbl_ovrd=off  block_type=logical
  Register : xbsIndex_r4/Register  init=0  rst=off  en=off  dbl_ovrd=off  block_type=register
  extd_out : Outport
  wires:
  Register/1 -> Logical1/1, Logical3/2
  clr/1 -> Inverter/1
  Logical1/1 -> Logical2/2
  Logical2/1 -> Register/1
  Inverter/1 -> Logical1/2
  Logical3/1 -> extd_out/1
  pulse_in/1 -> Logical3/1, Logical2/1

== system ddc_bpm_476_066/monit_pos_1/Cast1 ==
  data_in : Inport
  en : Inport  Port=2
  Register : xbsIndex_r4/Register  init=0  rst=off  en=on  dbl_ovrd=off  block_type=register
      settings: xl_area=[0, 0, 0, 0, 0, 0, 0]  block_version=VER_STRING_GOES_HERE
  Register1 : xbsIndex_r4/Register  init=0  rst=off  en=off  dbl_ovrd=off  block_type=register
      settings: xl_area=[0, 0, 0, 0, 0, 0, 0]  block_version=VER_STRING_GOES_HERE
  format1 : Subsystem
  out : Outport
  vld_out : Outport  Port=2
  wires:
  format1/1(dout) -> Register/1
  Register/1 -> out/1
  data_in/1 -> format1/1(din)
  Register1/1 -> vld_out/1
  en/1 -> Register1/1, Register/2

== system ddc_bpm_476_066/monit_pos_1/TDDM_monit_pos_1_out ==
  monit_pos_1_din : Inport
  monit_pos_1_ch_in : Inport  Port=2
  TDDM_monit_pos_1_out_int : Subsystem
  Terminator : Terminator
  monit_pos_1_x_out : Outport
  monit_pos_1_y_out : Outport  Port=2
  monit_pos_1_q_out : Outport  Port=3
  monit_pos_1_sum_out : Outport  Port=4
  wires:
  TDDM_monit_pos_1_out_int/1(dout_ch0) -> monit_pos_1_x_out/1
  TDDM_monit_pos_1_out_int/2(dout_ch1) -> monit_pos_1_y_out/1
  TDDM_monit_pos_1_out_int/3(dout_ch2) -> monit_pos_1_q_out/1
  TDDM_monit_pos_1_out_int/4(dout_ch3) -> monit_pos_1_sum_out/1
  monit_pos_1_din/1 -> TDDM_monit_pos_1_out_int/1(din)
  monit_pos_1_ch_in/1 -> TDDM_monit_pos_1_out_int/2(ch_in)
  TDDM_monit_pos_1_out_int/5(ch_out) -> Terminator/1

== system ddc_bpm_476_066/DDS_sub/TDM_dds_ch01_cosine/ST1 ==
  In : Inport
  Display : Display
  Sample Time : xbsIndex_r4/Sample Time  block_type=sampletime
      settings: infoedit="The Sample Time block reports the normalized sample period of its input.  A signal's normalized sample period is not equivalent to its Simulink absolute sample period.<br><br>Hardware notes: This block is implemented as a constant in hardware."
  X_monit1 : xbsIndex_r4/Gateway Out  inherit_from_input=on  hdl_port=off  timing_constraint=Data Rate  locs_specified=off  LOCs={}  UseAsDAC=off  DACChannel='1'  block_type=gatewayout
      settings: infoedit="Gateway out block.  Converts Xilinx fixed-point or floating-point type inputs into ouputs of type Simulink integer, single, double, or fixed point.<br><br>Hardware notes:  In hardware these blocks become top level output ports or are discarded, depending on how they are configured."
  wires:
  X_monit1/1 -> Display/1
  Sample Time/1 -> X_monit1/1
  In/1 -> Sample Time/1

== system ddc_bpm_476_066/DDS_sub/TDM_dds_ch01_cosine/ST2 ==
  In : Inport
  Display : Display
  Sample Time : xbsIndex_r4/Sample Time  block_type=sampletime
      settings: infoedit="The Sample Time block reports the normalized sample period of its input.  A signal's normalized sample period is not equivalent to its Simulink absolute sample period.<br><br>Hardware notes: This block is implemented as a constant in hardware."
  X_monit1 : xbsIndex_r4/Gateway Out  inherit_from_input=on  hdl_port=off  timing_constraint=Data Rate  locs_specified=off  LOCs={}  UseAsDAC=off  DACChannel='1'  block_type=gatewayout
      settings: infoedit="Gateway out block.  Converts Xilinx fixed-point or floating-point type inputs into ouputs of type Simulink integer, single, double, or fixed point.<br><br>Hardware notes:  In hardware these blocks become top level output ports or are discarded, depending on how they are configured."
  wires:
  X_monit1/1 -> Display/1
  Sample Time/1 -> X_monit1/1
  In/1 -> Sample Time/1

== system ddc_bpm_476_066/DDS_sub/TDM_dds_ch01_cosine/ST3 ==
  In : Inport
  Display : Display
  Sample Time : xbsIndex_r4/Sample Time  block_type=sampletime
      settings: infoedit="The Sample Time block reports the normalized sample period of its input.  A signal's normalized sample period is not equivalent to its Simulink absolute sample period.<br><br>Hardware notes: This block is implemented as a constant in hardware."
  X_monit1 : xbsIndex_r4/Gateway Out  inherit_from_input=on  hdl_port=off  timing_constraint=Data Rate  locs_specified=off  LOCs={}  UseAsDAC=off  DACChannel='1'  block_type=gatewayout
      settings: infoedit="Gateway out block.  Converts Xilinx fixed-point or floating-point type inputs into ouputs of type Simulink integer, single, double, or fixed point.<br><br>Hardware notes:  In hardware these blocks become top level output ports or are discarded, depending on how they are configured."
  wires:
  X_monit1/1 -> Display/1
  Sample Time/1 -> X_monit1/1
  In/1 -> Sample Time/1

== system ddc_bpm_476_066/DDS_sub/TDM_dds_ch01_cosine/ST5 ==
  In : Inport
  Display : Display
  Sample Time : xbsIndex_r4/Sample Time  block_type=sampletime
      settings: infoedit="The Sample Time block reports the normalized sample period of its input.  A signal's normalized sample period is not equivalent to its Simulink absolute sample period.<br><br>Hardware notes: This block is implemented as a constant in hardware."
  out : xbsIndex_r4/Gateway Out  inherit_from_input=on  hdl_port=off  timing_constraint=Data Rate  locs_specified=off  LOCs={}  UseAsDAC=off  DACChannel='1'  block_type=gatewayout
      settings: infoedit="Gateway out block.  Converts Xilinx fixed-point or floating-point type inputs into ouputs of type Simulink integer, single, double, or fixed point.<br><br>Hardware notes:  In hardware these blocks become top level output ports or are discarded, depending on how they are configured."
  wires:
  out/1 -> Display/1
  Sample Time/1 -> out/1
  In/1 -> Sample Time/1

== system ddc_bpm_476_066/DDS_sub/TDM_dds_ch01_sine/ST1 ==
  In : Inport
  Display : Display
  Sample Time : xbsIndex_r4/Sample Time  block_type=sampletime
      settings: infoedit="The Sample Time block reports the normalized sample period of its input.  A signal's normalized sample period is not equivalent to its Simulink absolute sample period.<br><br>Hardware notes: This block is implemented as a constant in hardware."
  X_monit1 : xbsIndex_r4/Gateway Out  inherit_from_input=on  hdl_port=off  timing_constraint=Data Rate  locs_specified=off  LOCs={}  UseAsDAC=off  DACChannel='1'  block_type=gatewayout
      settings: infoedit="Gateway out block.  Converts Xilinx fixed-point or floating-point type inputs into ouputs of type Simulink integer, single, double, or fixed point.<br><br>Hardware notes:  In hardware these blocks become top level output ports or are discarded, depending on how they are configured."
  wires:
  X_monit1/1 -> Display/1
  Sample Time/1 -> X_monit1/1
  In/1 -> Sample Time/1

== system ddc_bpm_476_066/DDS_sub/TDM_dds_ch01_sine/ST2 ==
  In : Inport
  Display : Display
  Sample Time : xbsIndex_r4/Sample Time  block_type=sampletime
      settings: infoedit="The Sample Time block reports the normalized sample period of its input.  A signal's normalized sample period is not equivalent to its Simulink absolute sample period.<br><br>Hardware notes: This block is implemented as a constant in hardware."
  X_monit1 : xbsIndex_r4/Gateway Out  inherit_from_input=on  hdl_port=off  timing_constraint=Data Rate  locs_specified=off  LOCs={}  UseAsDAC=off  DACChannel='1'  block_type=gatewayout
      settings: infoedit="Gateway out block.  Converts Xilinx fixed-point or floating-point type inputs into ouputs of type Simulink integer, single, double, or fixed point.<br><br>Hardware notes:  In hardware these blocks become top level output ports or are discarded, depending on how they are configured."
  wires:
  X_monit1/1 -> Display/1
  Sample Time/1 -> X_monit1/1
  In/1 -> Sample Time/1
